simulink library "Lib_PB_Battery_TMATS"  (R2017b)
settings: Solver=ode45  StartTime=0.0  StopTime=10.0  RelTol=1e-3  EnableMultiTasking=on
undefined symbols (not defined in the file): A, B, K, Q, R
libraries: Lib_PF_BusLoadDC_TMATS x1
Description:
  | Thomas Modules
settings Model: Creator=jwchapm2  LastModifiedBy=mebell
settings DataIOCC: LimitDataPoints=on  SaveFormat=Array
settings OptimizationCC: ExpressionDepthLimit=2147483647  LifeSpan=inf
settings DebuggingCC: UnderspecifiedInitializationDetection=Classic  MergeDetectMultiDrivingBlocksExec=none  SolverPrmCheckMsg=warning  StateNameClashWarn=warning  SFUnexpectedBacktrackingDiag=warning  SFNoUnconditionalDefaultTransitionDiag=warning  SFExecutionAtInitializationDiag=none
settings HardwareCC: ProdBitPerPointer=32  ProdBitPerSizeT=32  ProdBitPerPtrDiffT=32  ProdLargestAtomicFloat=None  ProdIntDivRoundTo=Undefined  ProdEndianess=Unspecified  ProdWordSize=32  ProdHWDeviceType=32-bit Generic
settings ModelReferenceCC: PropagateSignalLabelsOutOfModel=off
settings CodeAppCC: StateflowObjectComments=on
settings GRTTargetCC: TargetLangStandard=C89/C90 (ANSI)  GeneratePreprocessorConditionals=Disable all
settings ConfigComp: CovMetricSettings=dw  CovHtmlReporting=on  CovSaveCumulativeToWorkspaceVar=on  CovSaveSingleToWorkspaceVar=on  CovExternalEMLEnable=off

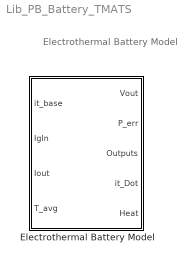
== system Lib_PB_Battery_TMATS ==
  note: Electrothermal
      | Battery Model
  "Electrothermal Battery Model " : Subsystem  mask(HiFiBattery){E0_M=3.3, Q_M=Q, R_M=R, K_M=K, B_M=B, SOC_Init_M=100.0, A_M=A, battery_type_M=Li-Ion, TempIn=Celsius}
      mask prompts: E0_M "E0_M – battery constant voltage (V)"; Q_M "Q_M – battery capacity (Ah)"; R_M "R_M – battery internal resistance (ohm)"; K_M "K_M – polarization constant (Ah^-1)"; B_M "B_M – exponential zone time constant inverse (Ah^-1)"; SOC_Init_M "SOC_Init_M – initial percentage state of charge (%)"; A_M "A_M – exponential zone amplitude (V)"; battery_type_M "battery_type_M - Li-Ion-, Ni-MH-, or Lead Acid-based chemistry"; TempIn "Input Temp Units:"
      mask help: This block represents a physics-based battery model. The output voltage is a function of the current drawn from the battery ('Iout'), and the time integral of the current drawn from the battery, ('it', in Amp-hours). You need an integrator that takes in it_dot, and you need to feed that integrated it value into it_base. The initial condition for it_base should be zero, as this integrator should keep track of consumed charge, in amp-hours. If you put in a value other than 100% for SOC_Init_M, then you will see a difference between the it_base (which always starts at zero), and it as you get it from the Outputs structure, which accounts for the difference in SOC_Init_M from 100%.
      mask init:
      | %Get current block name
      | block = gcb;
      | 
      | %Block under the mask(T_in inport)
      | block2 = [block '/T_avg'];
      | %Set T_in unit parameter to correct unit.
      | switch TempIn
      |     case 1 
      |         set_param(block2,'Unit','degF');
      |     case 2
      |         set_param(block2,'Unit','degC');
      |     case 3
      |         set_param(block2,'Unit','degR');
      |     case 4
      |         set_param(block2,'Unit','K');
      | end
      mask TypeOptions battery_type_M: Li-Ion | Ni-MH/Lead Acid
      mask TypeOptions TempIn: Fahrenheit | Celsius | Rankine | Kelvin
      mask DialogControl TempGroupVar Prompt: Temperature Units
      mask Display:
      | switch TempIn
      |     case 1
      |         port_label('input', 4, 'T_avg (F)');
      |     case 2
      |         port_label('input', 4, 'T_avg (C)');
      |     case 3
      |         port_label('input', 4, 'T_avg (Ra)');
      |     case 4
      |         port_label('input', 4, 'T_avg (K)');
      | end
      | port_label('input', 1, 'it_base');
      | port_label('input', 2, 'Igin');
      | port_label('input', 3, 'Iout');
      | port_label('output', 1, 'Vout');
      | port_label('output', 2, 'P_err');
      | port_label('output', 3, 'Outputs');
      | port_label('output', 4, 'it_Dot');
      | port_label('output', 5, 'Heat');

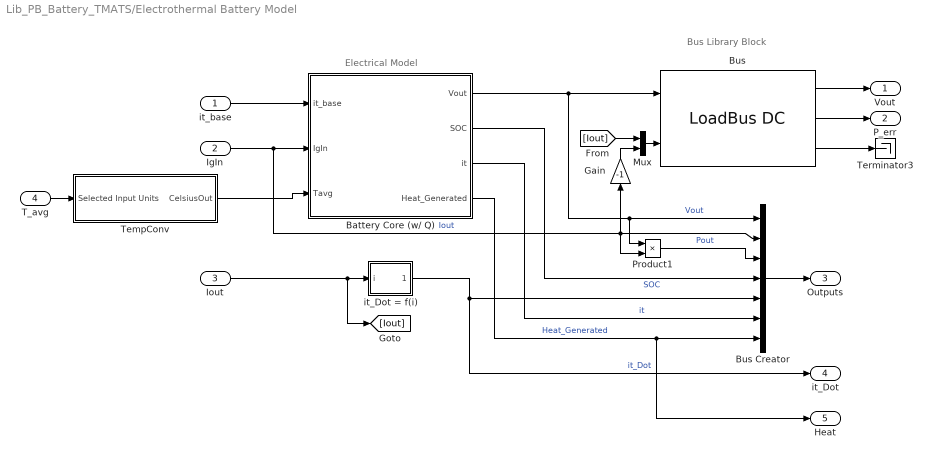
== system Lib_PB_Battery_TMATS/Electrothermal Battery Model  ==
  note: Bus Library Block
  note: Electrical Model
  it_base : Inport
  IgIn : Inport  Port=2
  Iout : Inport  Port=3
  T_avg : Inport  Port=4  Unit=degC
  Battery Core (w/ Q) : Subsystem
  Bus : Lib_PF_BusLoadDC_TMATS/LoadBus DC  PeInEN_M=off  P_M=0  BlkNm_M=double(gcb)
  Bus Creator : BusCreator  Inputs=7
  Gain : Gain  Gain=-1
  Mux : Mux  Inputs=2
  Product1 : Product
  "TempConv " : Subsystem  AncestorBlock=Lib_PB_BuckConv_TMATS/Buck Converter/TempConv
      mask DialogControl DescTextVar Prompt: Temperature Unit Converter
  Terminator3 : Terminator
  it_Dot = f(i) : Subsystem
  Vout : Outport
  P_err : Outport  Port=2
  Outputs : Outport  Port=3
  it_Dot : Outport  Port=4
  Heat : Outport  Port=5
  wires:
  Battery Core (w/ Q)/4(Heat_Generated) -> Bus Creator/7, Heat/1  "Heat_Generated"
  Bus Creator/1 -> Outputs/1
  IgIn/1 -> Bus Creator/2, Product1/2, Gain/1, Battery Core (w/ Q)/2(IgIn)  "Iout"
  it_Dot = f(i)/1(it_Dot) -> it_Dot/1, Bus Creator/5  "it_Dot"
  Mux/1 -> Bus/2
  Bus/1 -> Vout/1
  Iout/1 -> [Iout], it_Dot = f(i)/1(i)
  Bus/3 -> Terminator3/1
  Bus/2 -> P_err/1
  Gain/1 -> Mux/2
  [Iout] -> Mux/1
  Product1/1 -> Bus Creator/3  "Pout"
  Battery Core (w/ Q)/1(Vout) -> Bus/1, Product1/1, Bus Creator/1  "Vout"
  it_base/1 -> Battery Core (w/ Q)/1(it_base)
  Battery Core (w/ Q)/2(SOC) -> Bus Creator/4  "SOC"
  Battery Core (w/ Q)/3(it) -> Bus Creator/6  "it"
  T_avg/1 -> "TempConv "/1(Selected Input Units)
  "TempConv "/1(CelsiusOut) -> Battery Core (w/ Q)/3(Tavg)

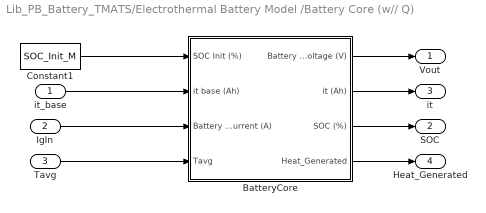
== system Lib_PB_Battery_TMATS/Electrothermal Battery Model /Battery Core (w// Q) ==
  it_base : Inport
  IgIn : Inport  Port=2
  Tavg : Inport  Port=3
  BatteryCore : Subsystem
  Constant1 : Constant  Value=SOC_Init_M
  Vout : Outport
  SOC : Outport  Port=2
  it : Outport  Port=3
  Heat_Generated : Outport  Port=4
  wires:
  BatteryCore/4(Heat_Generated) -> Heat_Generated/1
  BatteryCore/3(SOC (%)) -> SOC/1
  BatteryCore/1(Battery Voltage (V)) -> Vout/1
  BatteryCore/2(it (Ah)) -> it/1
  it_base/1 -> BatteryCore/2("it base (Ah) ")
  Tavg/1 -> BatteryCore/4("Tavg ")
  Constant1/1 -> BatteryCore/1("SOC Init (%) ")
  IgIn/1 -> BatteryCore/3("Battery Current (A) ")

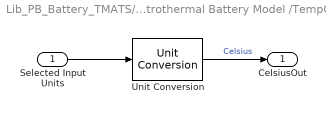
== system Lib_PB_Battery_TMATS/Electrothermal Battery Model /TempConv  ==
  Selected Input Units : Inport
  Unit Conversion : UnitConversion
  CelsiusOut : Outport  Unit=°C
  wires:
  Selected Input Units/1 -> Unit Conversion/1
  Unit Conversion/1 -> CelsiusOut/1  "Celsius"

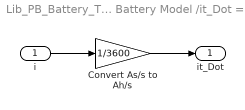
== system Lib_PB_Battery_TMATS/Electrothermal Battery Model /it_Dot = f(i) ==
  i : Inport
  Convert As/s to Ah/s : Gain  Gain=1/3600
  it_Dot : Outport
  wires:
  i/1 -> Convert As/s to Ah/s/1
  Convert As/s to Ah/s/1 -> it_Dot/1

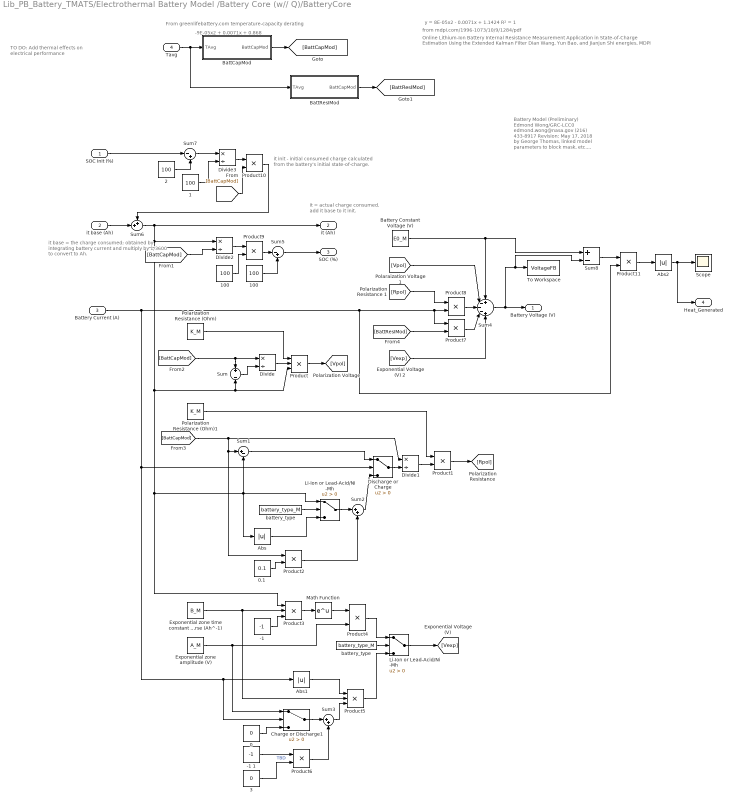
== system Lib_PB_Battery_TMATS/Electrothermal Battery Model /Battery Core (w// Q)/BatteryCore ==
  note: Online Lithium-Ion Battery Internal Resistance Measurement Application in State-of-Charge
      | Estimation Using the Extended Kalman Filter
      |
      | Dian Wang, Yun Bao, and Jianjun Shi
      |
      | energies, MDPI
  note: from mdpi.com/1996-1073/10/9/1284/pdf
  note: y = 8E-05x2 - 0.0071x + 1.1424 R² = 1
  note: From greenlifebattery.com temperature-capacity derating
  note: -9E-05x2 + 0.0071x + 0.868
  note: Battery Model (Preliminary)
      | Edmond Wong/GRC-LCC0
      | edmond.wong@nasa.gov
      | (216) 433-8917
      |
      | Revision: May 17, 2018
      | by George Thomas, linked model
      | parameters to block mask, etc.
      |
      | Revision: April 29, 2019
      | by Mark Bell
      | Heat output, initial temperature feedback
  note: it base = the charge consumed;
      | obtained by integrating battery current
      | and multiply by 1/3600 to convert to Ah.
  note: it init - initial consumed charge calculated
      | from the battery's initial state-of-charge.
  note: it = actual charge consumed.
      | add it base to it init.
  note: TO DO: Add thermal effects on electrical performance
  "SOC Init (%) " : Inport
  "it base (Ah) " : Inport  Port=2
  "Battery Current (A) " : Inport  Port=3
  "Tavg " : Inport  Port=4
  "-1 " : Constant  Value=-1
  -1 1 : Constant  Value=-1
  0 : Constant  Value=0
  0.1 : Constant  Value=0.1
  1 : Constant  Value=100
  100 : Constant  Value=100
  "100 " : Constant  Value=100
  2 : Constant  Value=100
  3 : Constant  Value=0
  Abs : Abs
  Abs1 : Abs
  Abs2 : Abs
  "BattCapMod " : Subsystem
  "BattResIMod " : Subsystem  AncestorBlock=Electrothermal_Battery_v1_LibraryBlockModel/Electrothermal Battery Model /Battery Core (w// Q)/BatteryCore/BattCapMod
  Battery Constant Voltage (V) : Constant  Value=E0_M
  Charge or Discharge1 : Switch  Criteria=u2 > Threshold
  Discharge or Charge : Switch  Criteria=u2 > Threshold
  Divide{,1..3} (4 alike) : Product  Inputs=*/
  Exponential zone amplitude (V) : Constant  Value=A_M
  Exponential zone time constant inverse (Ah^-1) : Constant  Value=B_M
  Li-Ion or Lead-Acid/Ni-Mh : Switch  Criteria=u2 > Threshold
  "Li-Ion or Lead-Acid/Ni-Mh " : Switch  Criteria=u2 > Threshold
  Math Function : Math  SaturateOnIntegerOverflow=on
  Polarization Resistance (Ohm) : Constant  Value=K_M
  Polarization Resistance (Ohm)1 : Constant  Value=K_M
  Product : Product  Inputs=3
  Product{1..2,4,6..11} (9 alike) : Product
  Product3 : Product  Inputs=3
  Product5 : Product  Inputs=3
  Scope : Scope
  Sum : Sum  Inputs=+||-
  Sum1 : Sum  Inputs=|+-
  Sum2 : Sum  Inputs=|++
  Sum3 : Sum  Inputs=|++
  Sum4 : Sum  Inputs=+---+
  Sum5 : Sum  Inputs=|-+
  Sum6 : Sum  Inputs=++|
  Sum7 : Sum  Inputs=|-+
  Sum8 : Sum  Inputs=+-
  To Workspace : ToWorkspace  VariableName=VoltageFB  SampleTime=-1
  battery_type : Constant  Value=battery_type_M
  "battery_type " : Constant  Value=battery_type_M
  Battery Voltage (V) : Outport
  it (Ah) : Outport  Port=2
  SOC (%) : Outport  Port=3
  Heat_Generated : Outport  Port=4
  wires:
  Sum4/1 -> Battery Voltage (V)/1, To Workspace/1, Sum8/2
  "Battery Current (A) "/1 -> Abs1/1, Charge or Discharge1/2, Discharge or Charge/2, Product7/1, Product8/2, Product11/2
  Battery Constant Voltage (V)/1 -> Sum4/1, Sum8/1
  Product11/1 -> Abs2/1
  Sum8/1 -> Product11/1
  Abs2/1 -> Scope/1, Heat_Generated/1
  Divide1/1 -> Product1/2
  Product1/1 -> [Rpol]
  0.1/1 -> Product2/2
  Sum3/1 -> Product5/3
  Li-Ion or Lead-Acid/Ni-Mh/1 -> Sum2/1
  Product3/1 -> Math Function/1
  Sum2/1 -> Discharge or Charge/3
  Exponential zone time constant inverse (Ah^-1)/1 -> Product3/2, Product5/2
  Abs/1 -> Li-Ion or Lead-Acid/Ni-Mh/3
  0/1 -> Charge or Discharge1/3
  Discharge or Charge/1 -> Divide1/2
  Abs1/1 -> Product5/1
  Product2/1 -> Sum2/2
  Polarization Resistance (Ohm)/1 -> Product/1
  "Li-Ion or Lead-Acid/Ni-Mh "/1 -> [Vexp]
  Sum5/1 -> SOC (%)/1
  Product4/1 -> "Li-Ion or Lead-Acid/Ni-Mh "/1
  [Vpol] -> Sum4/2
  Sum1/1 -> Discharge or Charge/1
  [Rpol] -> Product8/1
  -1 1/1 -> Product6/1
  Divide2/1 -> Product9/1
  Math Function/1 -> Product4/1
  Charge or Discharge1/1 -> Sum3/1
  "-1 "/1 -> Product3/3
  100/1 -> Product9/2
  [BattCapMod] -> Sum1/1, Product2/1, Divide1/1
  Sum6/1 -> it (Ah)/1, Product3/1, Abs/1, Li-Ion or Lead-Acid/Ni-Mh/1, Sum1/2, Sum/2, Product/3, Divide2/1
  Product6/1 -> Sum3/2
  "battery_type "/1 -> "Li-Ion or Lead-Acid/Ni-Mh "/2
  [Vexp] -> Sum4/5
  battery_type/1 -> Li-Ion or Lead-Acid/Ni-Mh/2
  Product8/1 -> Sum4/3
  3/1 -> Product6/2  "TBD"
  Exponential zone amplitude (V)/1 -> Charge or Discharge1/1, Product4/2
  Product7/1 -> Sum4/4
  Sum/1 -> Divide/2
  Product/1 -> [Vpol]
  Product5/1 -> "Li-Ion or Lead-Acid/Ni-Mh "/3
  Divide/1 -> Product/2
  Polarization Resistance (Ohm)1/1 -> Product1/1
  1/1 -> Divide3/2
  "it base (Ah) "/1 -> Sum6/2
  Product10/1 -> Sum6/1
  Sum7/1 -> Divide3/1
  2/1 -> Sum7/2
  "100 "/1 -> Sum5/2
  Divide3/1 -> Product10/1
  Product9/1 -> Sum5/1
  "SOC Init (%) "/1 -> Sum7/1
  "BattCapMod "/1(BattCapMod) -> [BattCapMod]
  [BattCapMod] -> Product10/2
  [BattCapMod] -> Divide2/2
  [BattCapMod] -> Sum/1, Divide/1
  "BattResIMod "/1(BattCapMod) -> [BattResIMod]
  "Tavg "/1 -> "BattResIMod "/1(TAvg), "BattCapMod "/1(TAvg)
  [BattResIMod] -> Product7/2

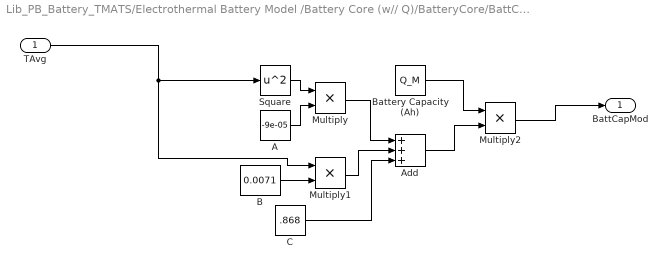
== system Lib_PB_Battery_TMATS/Electrothermal Battery Model /Battery Core (w// Q)/BatteryCore/BattCapMod  ==
  TAvg : Inport
  "A " : Constant  Value=-9e-05
  Add : Sum  Inputs=+++
  "B " : Constant  Value=0.0071
  Battery Capacity (Ah) : Constant  Value=Q_M
  C : Constant  Value=.868
  Multiply : Product
  Multiply1 : Product
  Multiply2 : Product
  Square : Math  Operator=square  SaturateOnIntegerOverflow=on
  BattCapMod : Outport
  wires:
  "B "/1 -> Multiply1/2
  Battery Capacity (Ah)/1 -> Multiply2/1
  TAvg/1 -> Multiply1/1, Square/1
  Square/1 -> Multiply/1
  Multiply/1 -> Add/1
  "A "/1 -> Multiply/2
  Add/1 -> Multiply2/2
  Multiply1/1 -> Add/2
  C/1 -> Add/3
  Multiply2/1 -> BattCapMod/1

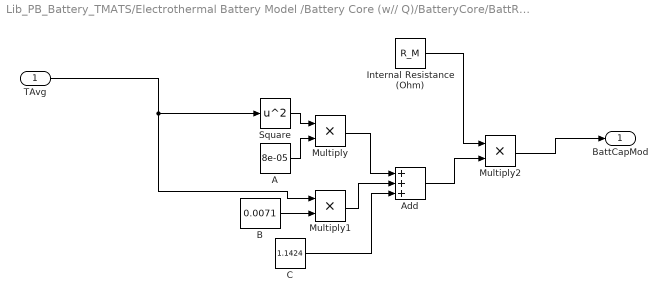
== system Lib_PB_Battery_TMATS/Electrothermal Battery Model /Battery Core (w// Q)/BatteryCore/BattResIMod  ==
  TAvg : Inport
  "A " : Constant  Value=8e-05
  Add : Sum  Inputs=+++
  "B " : Constant  Value=0.0071
  C : Constant  Value=1.1424
  Internal Resistance (Ohm) : Constant  Value=R_M
  Multiply : Product
  Multiply1 : Product
  Multiply2 : Product
  Square : Math  Operator=square  SaturateOnIntegerOverflow=on
  BattCapMod : Outport
  wires:
  "B "/1 -> Multiply1/2
  Internal Resistance (Ohm)/1 -> Multiply2/1
  TAvg/1 -> Multiply1/1, Square/1
  Square/1 -> Multiply/1
  Multiply/1 -> Add/1
  "A "/1 -> Multiply/2
  Add/1 -> Multiply2/2
  Multiply1/1 -> Add/2
  C/1 -> Add/3
  Multiply2/1 -> BattCapMod/1
